simulink model "Assignment_2_Final_Submission"  (R2022b)
settings: Solver=FixedStepAuto  StartTime=0.0  StopTime=10.0  FixedStep=1e-3  RelTol=1e-3  EnableMultiTasking=on
undefined symbols (not defined in the file): A0, A1, D0, D1, D10, D11, D12, D13, D2, D3, D4, D5, D6, D7, D8, D9, magnitude, PTA0, PTA1, PTA2, PTB2, PTB23, PTB3, PTB9, PTC16, PTC17, PTC2, PTC3, PTC4, PTD0, PTD1, PTD2, PTD3
libraries: frdmk64flib x19, etargetslib x8, simulink x2, dspstat3 x1
(part 1 of 2)
settings Model: ExtModeTrigDuration=5  Creator=annan  LastModifiedBy=danie
settings OptimizationCC: EnhancedBackFolding=on  PassReuseOutputArgsAs=Individual arguments  ZeroExternalMemoryAtStartup=off  ZeroInternalMemoryAtStartup=off  MaxStackSize=64  OptimizeBlockOrder=speed  DifferentSizesBufferReuse=on  OptimizationCustomize=off  EfficientTunableParamExpr=on
settings DebuggingCC: ParameterTunabilityLossMsg=error
settings HardwareCC: ProdBitPerPointer=32  ProdBitPerSizeT=32  ProdBitPerPtrDiffT=32  ProdLargestAtomicInteger=Long  ProdLargestAtomicFloat=Double  ProdWordSize=32  ProdHWDeviceType=ARM Compatible->ARM Cortex
settings SFSimCC: MATLABDynamicMemAlloc=off
settings RTWCC: Description=Embedded Coder  SystemTargetFile=ert.tlc  HardwareBoard=NXP FRDM-K64F  TLCOptions="-aInlineSetEventsForThisBaseRateFcn=TLC_FALSE -aSuppressMultiTaskScheduler=TLC_FALSE  -aRateBasedStepFcn=0"  TemplateMakefile=ert_default_tmf  Toolchain=GNU Tools for ARM Embedded Processors
settings CodeAppCC: ForceParamTrailComments=on  IgnoreCustomStorageClasses=off  OperatorAnnotations=on  SimulinkDataObjDesc=on  SFDataObjDesc=on  InsertBlockDesc=on
settings ERTTargetCC: ExtModeTransport=4  ExtModeMexFile=sendToCommService

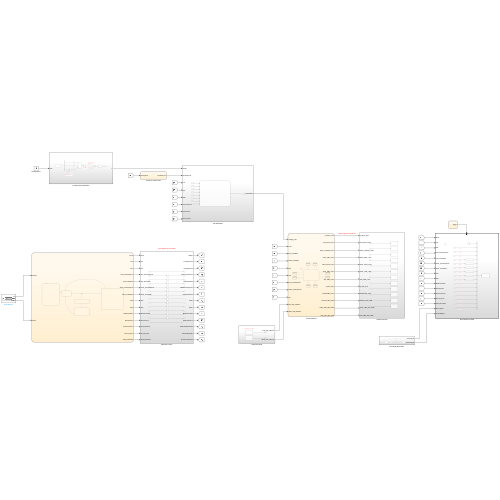
[thumbnail: Simulink's stored preview of the top-level diagram]
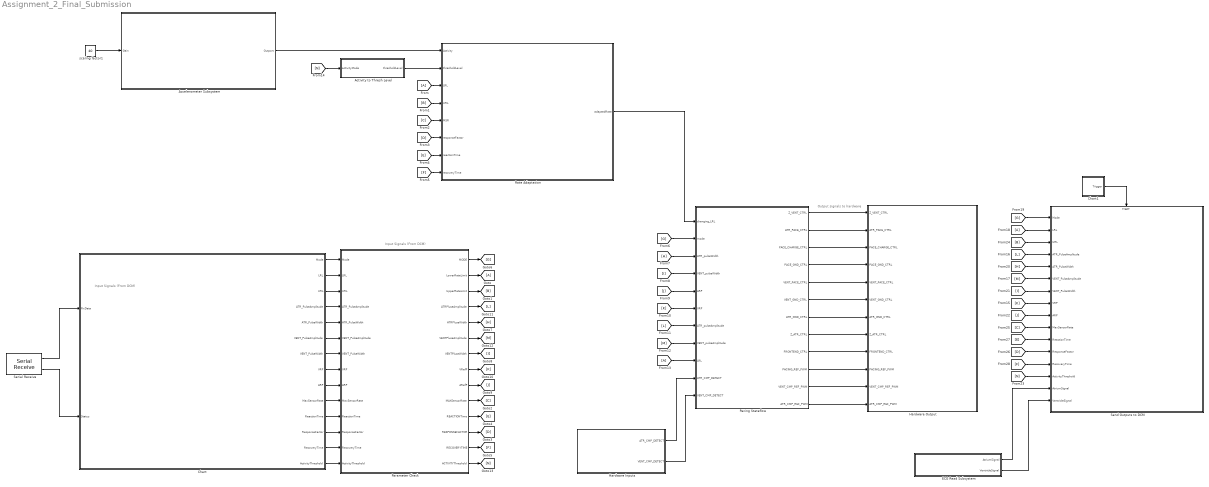
== system Assignment_2_Final_Submission ==
  note: Input Signals (From DCM)
  note: Output signals to hardware
  note: Input Signals (From DCM)
  Accelerometer Subsystem : Subsystem
  Activity to Thresh Level : Stateflow chart  TreatAsAtomicUnit=on
  Chart : Stateflow chart  TreatAsAtomicUnit=on
      settings: PortSchema="{\"entries\":[{\"content\":{\"sides\":[{\"content\":{\"connectorIds\":[\"In1\",\"In2\"]},\"type\":\"ConnectorPlacement.EquallySpacedRectSide\",\"uuid\":\"5dec20b2-4828-40f7-ab17-581616d768e4\"},{\"content\":{\"connectorIds\":[\"Out14\",\"Out1\",\"Out13\",\"Out12\",\"Out11\",\"Out10\",\"Out9\",\"Out8\",\"Out7\",\"Out6\",\"Out5\",\"Out4\",\"Out3\",\"Out2\"],\"side\":\"RIGHT\"},\"type\":\"ConnectorPlacement.EquallySpacedRectSide\",\"uuid\":\"fe0d7708-8c60-4078-b2a9-9a22708a989b\"},{\"content\":{\"connectorIds\":[],\"side\":\"TOP\"},\"type\":\"ConnectorPlacement.EquallySpacedRectSide\",\"uuid\":\"c8cd286c-7cc7-4d1d-92dd-859e210849b8\"},{\"content\":{\"connectorIds\":[],\"side\":\"BOTTOM\"},\"type\":\"ConnectorPlacement.EquallySpacedRectSide\",\"uuid\":\"bbfa5a44-a83c-4407-89b4-d26b2a8b5140\"}]},\"type\":\"ConnectorPlacement.EquallySpacedConnector\",\"uuid\":\"7f21e6d2-2aa6-491e-bb3e-ebcef11de234\"}],\"packageUris\":[\"http://schema.mathworks.com/mf0/Connector/R2020b\"],\"version\":\"1.0\"}"
  Chart1 : Stateflow chart  TreatAsAtomicUnit=on
  ECG Read Subsystem : Subsystem
  From : From
  From13 : From
  From18 : From
  Goto : Goto
  Hardware Inputs : Subsystem
  Hardware Output : Subsystem
  Pacing Stateflow : Stateflow chart  TreatAsAtomicUnit=on
      settings: PortSchema="{\"entries\":[{\"content\":{\"sides\":[{\"content\":{\"connectorIds\":[\"In1\",\"In2\",\"In3\",\"In4\",\"In6\",\"In5\",\"In9\",\"In8\",\"In7\",\"In10\",\"In11\"]},\"type\":\"ConnectorPlacement.EquallySpacedRectSide\",\"uuid\":\"576c6451-25f7-4bf9-8ba9-b62bfe0038eb\"},{\"content\":{\"connectorIds\":[\"Out1\",\"Out2\",\"Out3\",\"Out4\",\"Out5\",\"Out6\",\"Out7\",\"Out8\",\"Out9\",\"Out10\",\"Out11\",\"Out12\"],\"side\":\"RIGHT\"},\"type\":\"ConnectorPlacement.EquallySpacedRectSide\",\"uuid\":\"13f5cd1e-83b9-45c9-ae47-e36f7742cdf1\"},{\"content\":{\"connectorIds\":[],\"side\":\"TOP\"},\"type\":\"ConnectorPlacement.EquallySpacedRectSide\",\"uuid\":\"e0eaa1cf-7eb4-4233-8973-4ce0d50eac65\"},{\"content\":{\"connectorIds\":[],\"side\":\"BOTTOM\"},\"type\":\"ConnectorPlacement.EquallySpacedRectSide\",\"uuid\":\"d60b4a6c-f34d-471d-8156-20bbac3fd058\"}]},\"type\":\"ConnectorPlacement.EquallySpacedConnector\",\"uuid\":\"6190d1e8-de04-4ebf-bfa3-72cd0ed3652a\"}],\"packageUris\":[\"http://schema.mathworks.com/mf0/Connector/R2020b\"],\"version\":\"1.0\"}"
  Parameter Check : Subsystem
  Rate Adaptation : Subsystem
  Send Outputs to DCM : Subsystem
  Serial Receive : frdmk64flib/Serial Receive  SCIModule=0  Baudrate=uint32(9600)  Parity=None  StopBits=1  HardwareFlowControl=None  ByteOrder=LittleEndian  DataType=uint8  DataLength=29  BlockingMode=off  OutputStatus=on  SampleTime=-1
  scaling factor1 : Constant  Value=40
  wires:
  Pacing Stateflow/1(Z_VENT_CTRL) -> Hardware Output/1(Z_VENT_CTRL)
  Pacing Stateflow/2(ATR_PACE_CTRL) -> Hardware Output/2(ATR_PACE_CTRL)
  Pacing Stateflow/3(PACE_CHARGE_CTRL) -> Hardware Output/3(PACE_CHARGE_CTRL)
  Pacing Stateflow/4(PACE_GND_CTRL) -> Hardware Output/4(PACE_GND_CTRL)
  Pacing Stateflow/5(VENT_PACE_CTRL) -> Hardware Output/5(VENT_PACE_CTRL)
  Pacing Stateflow/6(VENT_GND_CTRL) -> Hardware Output/6(VENT_GND_CTRL)
  Pacing Stateflow/7(ATR_GND_CTRL) -> Hardware Output/7(ATR_GND_CTRL)
  Pacing Stateflow/8(Z_ATR_CTRL) -> Hardware Output/8(Z_ATR_CTRL)
  From13/1 -> Pacing Stateflow/7(LRL)
  [K] -> Pacing Stateflow/5(VRP)
  [H] -> Pacing Stateflow/3(ATR_pulseWidth)
  Pacing Stateflow/10(PACING_REF_PWM) -> Hardware Output/10(PACING_REF_PWM)
  [M] -> Pacing Stateflow/8(VENT_pulseAmplitude)
  Pacing Stateflow/9(FRONTEND_CTRL) -> Hardware Output/9(FRONTEND_CTRL)
  Pacing Stateflow/11(VENT_CMP_REF_PWM) -> Hardware Output/11(VENT_CMP_REF_PWM)
  Pacing Stateflow/12(ATR_CMP_REF_PWM) -> Hardware Output/12(ATR_CMP_REF_PWM)
  [I] -> Pacing Stateflow/4(VENT_pulseWidth)
  [J] -> Pacing Stateflow/6(ARP)
  [L] -> Pacing Stateflow/9(ATR_pulseAmplitude)
  [G] -> Pacing Stateflow/2(mode)
  [D] -> Rate Adaptation/6(responseFactor)
  [C] -> Rate Adaptation/5(MSR)
  [B] -> Rate Adaptation/4(URL)
  Activity to Thresh Level/1(thresholdLevel) -> Rate Adaptation/2(thresholdLevel)
  Accelerometer Subsystem/1(Outport) -> Rate Adaptation/1(Activity)
  [E] -> Rate Adaptation/7(reactionTime)
  [F] -> Rate Adaptation/8(recoveryTime)
  From/1 -> Rate Adaptation/3(LRL)
  scaling factor1/1 -> Accelerometer Subsystem/1(Gain)
  [N] -> Activity to Thresh Level/1(activityMode)
  Rate Adaptation/1(adaptedRate) -> Pacing Stateflow/1(changing_LRL)
  ECG Read Subsystem/2(VentricleSignal) -> Send Outputs to DCM/16(VentricleSignal)
  ECG Read Subsystem/1(AtriumSignal) -> Send Outputs to DCM/15(AtriumSignal)
  Chart1/1(Trigger) -> Send Outputs to DCM/Trigger
  Hardware Inputs/1(ATR_CMP_DETECT) -> Pacing Stateflow/10(ATR_CMP_DETECT)
  Hardware Inputs/2(VENT_CMP_DETECT) -> Pacing Stateflow/11(VENT_CMP_DETECT)
  Parameter Check/2(LowerRateLimit) -> Goto/1
  Parameter Check/3(UpperRateLimit) -> [B]
  Parameter Check/10(MAXSensorRate) -> [C]
  Parameter Check/12(RESPONSEFACTOR) -> [D]
  Parameter Check/11(REACTIONTime) -> [E]
  Parameter Check/13(RECOVERYTIME) -> [F]
  Parameter Check/1(MODE) -> [G]
  Parameter Check/5(ATRPluseWidth) -> [H]
  Parameter Check/7(VENTPluseWidth) -> [I]
  Parameter Check/9(ARefP) -> [J]
  Parameter Check/8(VRefP) -> [K]
  Parameter Check/4(ATRPluseAmplitude) -> [L]
  Parameter Check/6(VENTPluseAmplitude) -> [M]
  Parameter Check/14(ACTIVITYThreshold) -> [N]
  From18/1 -> Send Outputs to DCM/2(LRL)
  [B] -> Send Outputs to DCM/3(URL)
  [L] -> Send Outputs to DCM/4(ATR_PulseAmplitude)
  [H] -> Send Outputs to DCM/5(ATR_PulseWidth)
  [M] -> Send Outputs to DCM/6(VENT_PulseAmplitude)
  [I] -> Send Outputs to DCM/7(VENT_PulseWidth)
  [G] -> Send Outputs to DCM/1(Mode)
  [K] -> Send Outputs to DCM/8(VRP)
  [J] -> Send Outputs to DCM/9(ARP)
  [C] -> Send Outputs to DCM/10(MaxSensorRate)
  [E] -> Send Outputs to DCM/11(ReactionTime)
  [F] -> Send Outputs to DCM/13(RecoveryTime)
  [D] -> Send Outputs to DCM/12(ResponseFactor)
  Chart/3(RecoveryTime) -> Parameter Check/13("RecoveryTime ")
  Chart/2(ActivityThreshold) -> Parameter Check/14("ActivityThreshold ")
  Chart/7(ARP) -> Parameter Check/9(ARP)
  Chart/10(VENT_PulseAmplitude) -> Parameter Check/6("VENT_PulseAmplitude ")
  Chart/11(ATR_PulseWidth) -> Parameter Check/5("ATR_PulseWidth ")
  Chart/9(VENT_PulseWidth) -> Parameter Check/7("VENT_PulseWidth ")
  Chart/5(ReactionTime) -> Parameter Check/11("ReactionTime ")
  Chart/1(LRL) -> Parameter Check/2(LRL)
  Chart/14(Mode) -> Parameter Check/1(Mode)
  Serial Receive/2 -> Chart/2(Status)
  Serial Receive/1 -> Chart/1(RxData)
  Chart/6(MaxSensorRate) -> Parameter Check/10("MaxSensorRate ")
  Chart/12(ATR_PulseAmplitude) -> Parameter Check/4("ATR_PulseAmplitude ")
  Chart/8(VRP) -> Parameter Check/8(VRP)
  Chart/13(URL) -> Parameter Check/3(URL)
  Chart/4(ResponseFactor) -> Parameter Check/12("ResponseFactor ")
  [N] -> Send Outputs to DCM/14(ActivityThreshold)

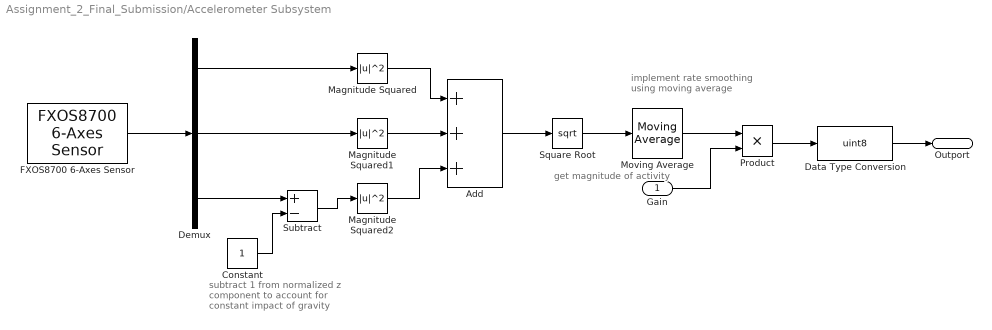
== system Assignment_2_Final_Submission/Accelerometer Subsystem ==
  note: subtract 1 from normalized z component to account for constant impact of gravity
  note: get magnitude of activity
  note: implement rate smoothing using moving average
  Gain : Inport
  Add : Sum  Inputs=+++  OutDataTypeStr=single
  Constant : Constant
  Data Type Conversion : DataTypeConversion  OutDataTypeStr=uint8  SaturateOnIntegerOverflow=off  RndMeth=Floor
  Demux : Demux  Outputs=3
  FXOS8700 6-Axes Sensor : frdmk64flib/FXOS8700 6-Axes Sensor  Activesensor=Accelerometer only  ODR=800Hz  HybridODR=400Hz  Accelfullrange=-4g to +4g  SampleTime=-1
  Magnitude Squared : Math  Operator=magnitude^2  OutDataTypeStr=single
  Magnitude Squared1 : Math  Operator=magnitude^2  OutDataTypeStr=single
  Magnitude Squared2 : Math  Operator=magnitude^2  OutDataTypeStr=single
  Moving Average : dspstat3/Moving Average  Method=Sliding window  ForgettingFactorPort=off  SpecifyWindowLength=on  WindowLength=1  OverlapLength=0  AllowArbitraryInputLength=off  ForgettingFactor=0.9  SimulateUsing=Code generation
  Product : Product
  Square Root : Sqrt  OutDataTypeStr=single
  Subtract : Sum  Inputs=+-
  Outport : Outport  OutDataTypeStr=uint8
  wires:
  FXOS8700 6-Axes Sensor/1 -> Demux/1
  Demux/2 -> Magnitude Squared1/1
  Demux/1 -> Magnitude Squared/1
  Demux/3 -> Subtract/1
  Magnitude Squared2/1 -> Add/3
  Magnitude Squared/1 -> Add/1
  Magnitude Squared1/1 -> Add/2
  Add/1 -> Square Root/1
  Constant/1 -> Subtract/2
  Subtract/1 -> Magnitude Squared2/1
  Square Root/1 -> Moving Average/1
  Gain/1 -> Product/2
  Product/1 -> Data Type Conversion/1
  Data Type Conversion/1 -> Outport/1
  Moving Average/1 -> Product/1

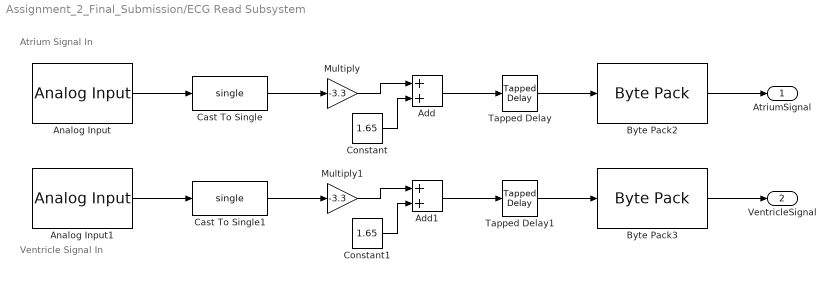
== system Assignment_2_Final_Submission/ECG Read Subsystem ==
  note: Ventricle Signal In
  note: Atrium Signal In
  Add : Sum
  Add1 : Sum
  Analog Input : frdmk64flib/Analog Input  Whichpin=PTB2 (A0)  SampleTime=0.002
  Analog Input1 : frdmk64flib/Analog Input  Whichpin=PTB3 (A1)  SampleTime=0.002
  Byte Pack2 : etargetslib/Byte Pack  datatypes={'single'}  byteAlign=1
  Byte Pack3 : etargetslib/Byte Pack  datatypes={'single'}  byteAlign=1
  Cast To Single : DataTypeConversion  OutDataTypeStr=single  SaturateOnIntegerOverflow=off  RndMeth=Floor
  Cast To Single1 : DataTypeConversion  OutDataTypeStr=single  SaturateOnIntegerOverflow=off  RndMeth=Floor
  Constant : Constant  Value=1.65  OutDataTypeStr=single
  Constant1 : Constant  Value=1.65  OutDataTypeStr=single
  Multiply : Gain  Gain=-3.3
  Multiply1 : Gain  Gain=-3.3
  Tapped Delay : simulink/Discrete/Tapped Delay  vinit=0.0  samptime=-1  NumDelays=9  DelayOrder=Oldest  includeCurrent=on
  Tapped Delay1 : simulink/Discrete/Tapped Delay  vinit=0.0  samptime=-1  NumDelays=9  DelayOrder=Oldest  includeCurrent=on
  AtriumSignal : Outport
  VentricleSignal : Outport  Port=2
  wires:
  Tapped Delay/1 -> Byte Pack2/1
  Cast To Single1/1 -> Multiply1/1
  Cast To Single/1 -> Multiply/1
  Analog Input/1 -> Cast To Single/1
  Tapped Delay1/1 -> Byte Pack3/1
  Analog Input1/1 -> Cast To Single1/1
  Byte Pack2/1 -> AtriumSignal/1
  Byte Pack3/1 -> VentricleSignal/1
  Add/1 -> Tapped Delay/1
  Multiply/1 -> Add/1
  Constant/1 -> Add/2
  Multiply1/1 -> Add1/1
  Add1/1 -> Tapped Delay1/1
  Constant1/1 -> Add1/2

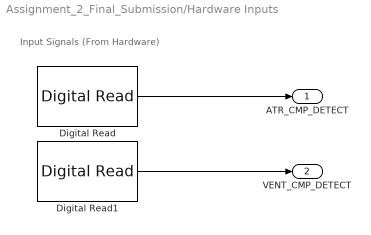
== system Assignment_2_Final_Submission/Hardware Inputs ==
  note: Input Signals (From Hardware)
  Digital Read : frdmk64flib/Digital Read  Whichpin=PTC16 (D0)  SampleTime=-1
  Digital Read1 : frdmk64flib/Digital Read  Whichpin=PTC17 (D1)  SampleTime=-1
  ATR_CMP_DETECT : Outport
  VENT_CMP_DETECT : Outport  Port=2
  wires:
  Digital Read/1 -> ATR_CMP_DETECT/1
  Digital Read1/1 -> VENT_CMP_DETECT/1

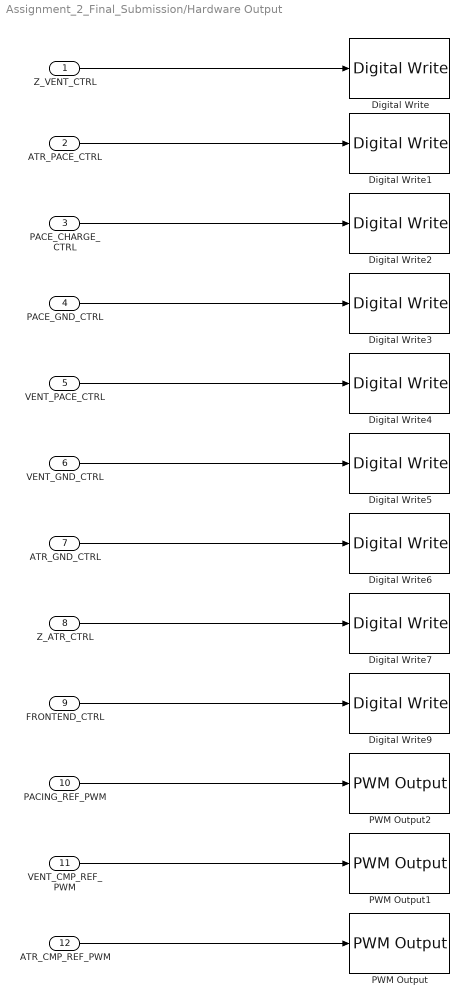
== system Assignment_2_Final_Submission/Hardware Output ==
  Z_VENT_CTRL : Inport
  ATR_PACE_CTRL : Inport  Port=2
  PACE_CHARGE_CTRL : Inport  Port=3
  PACE_GND_CTRL : Inport  Port=4
  VENT_PACE_CTRL : Inport  Port=5
  VENT_GND_CTRL : Inport  Port=6
  ATR_GND_CTRL : Inport  Port=7
  Z_ATR_CTRL : Inport  Port=8
  FRONTEND_CTRL : Inport  Port=9
  PACING_REF_PWM : Inport  Port=10
  VENT_CMP_REF_PWM : Inport  Port=11
  ATR_CMP_REF_PWM : Inport  Port=12
  Digital Write : frdmk64flib/Digital Write  Whichpin=PTC3 (D7)
  Digital Write1 : frdmk64flib/Digital Write  Whichpin=PTA0 (D8)
  Digital Write2 : frdmk64flib/Digital Write  Whichpin=PTB9 (D2)
  Digital Write3 : frdmk64flib/Digital Write  Whichpin=PTD0 (D10)
  Digital Write4 : frdmk64flib/Digital Write  Whichpin=PTC4 (D9)
  Digital Write5 : frdmk64flib/Digital Write  Whichpin=PTD3 (D12)
  Digital Write6 : frdmk64flib/Digital Write  Whichpin=PTD2 (D11)
  Digital Write7 : frdmk64flib/Digital Write  Whichpin=PTB23 (D4)
  Digital Write9 : frdmk64flib/Digital Write  Whichpin=PTD1 (D13)
  PWM Output : frdmk64flib/PWM Output  Whichpin=PTC2 (D6)  InitialFrequency=2000  InitialDutyCycle=0
  PWM Output1 : frdmk64flib/PWM Output  Whichpin=PTA1 (D3)  InitialFrequency=2000  InitialDutyCycle=0
  PWM Output2 : frdmk64flib/PWM Output  Whichpin=PTA2 (D5)  InitialFrequency=2000  InitialDutyCycle=0
  wires:
  Z_VENT_CTRL/1 -> Digital Write/1
  ATR_PACE_CTRL/1 -> Digital Write1/1
  PACE_CHARGE_CTRL/1 -> Digital Write2/1
  PACE_GND_CTRL/1 -> Digital Write3/1
  VENT_PACE_CTRL/1 -> Digital Write4/1
  VENT_GND_CTRL/1 -> Digital Write5/1
  ATR_GND_CTRL/1 -> Digital Write6/1
  Z_ATR_CTRL/1 -> Digital Write7/1
  PACING_REF_PWM/1 -> PWM Output2/1
  FRONTEND_CTRL/1 -> Digital Write9/1
  VENT_CMP_REF_PWM/1 -> PWM Output1/1
  ATR_CMP_REF_PWM/1 -> PWM Output/1

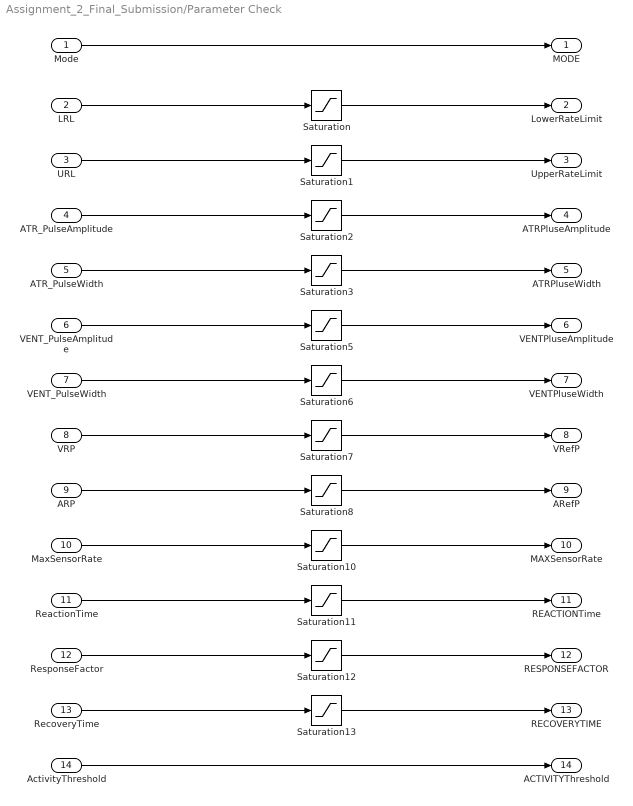
== system Assignment_2_Final_Submission/Parameter Check ==
  Mode : Inport
  LRL : Inport  Port=2
  URL : Inport  Port=3
  "ATR_PulseAmplitude " : Inport  Port=4  OutDataTypeStr=single
  "ATR_PulseWidth " : Inport  Port=5
  "VENT_PulseAmplitude " : Inport  Port=6
  "VENT_PulseWidth " : Inport  Port=7
  VRP : Inport  Port=8
  ARP : Inport  Port=9
  "MaxSensorRate " : Inport  Port=10
  "ReactionTime " : Inport  Port=11
  "ResponseFactor " : Inport  Port=12
  "RecoveryTime " : Inport  Port=13
  "ActivityThreshold " : Inport  Port=14
  Saturation : Saturate  UpperLimit=175  LowerLimit=30
  Saturation1 : Saturate  UpperLimit=175  LowerLimit=60
  Saturation10 : Saturate  UpperLimit=175  LowerLimit=50
  Saturation11 : Saturate  UpperLimit=50  LowerLimit=10
  Saturation12 : Saturate  UpperLimit=16  LowerLimit=1
  Saturation13 : Saturate  UpperLimit=16  LowerLimit=2
  Saturation2 : Saturate  UpperLimit=5  LowerLimit=0.5
  Saturation3 : Saturate  UpperLimit=1.9  LowerLimit=0.05
  Saturation5 : Saturate  UpperLimit=5  LowerLimit=0.5
  Saturation6 : Saturate  UpperLimit=1.9  LowerLimit=0.05
  Saturation7 : Saturate  UpperLimit=500  LowerLimit=150
  Saturation8 : Saturate  UpperLimit=500  LowerLimit=150
  MODE : Outport
  LowerRateLimit : Outport  Port=2
  UpperRateLimit : Outport  Port=3
  ATRPluseAmplitude : Outport  Port=4  OutDataTypeStr=single
  ATRPluseWidth : Outport  Port=5
  VENTPluseAmplitude : Outport  Port=6
  VENTPluseWidth : Outport  Port=7
  VRefP : Outport  Port=8
  ARefP : Outport  Port=9
  MAXSensorRate : Outport  Port=10
  REACTIONTime : Outport  Port=11
  RESPONSEFACTOR : Outport  Port=12
  RECOVERYTIME : Outport  Port=13
  ACTIVITYThreshold : Outport  Port=14
  wires:
  LRL/1 -> Saturation/1
  Saturation/1 -> LowerRateLimit/1
  Saturation1/1 -> UpperRateLimit/1
  URL/1 -> Saturation1/1
  Mode/1 -> MODE/1
  "ATR_PulseAmplitude "/1 -> Saturation2/1
  Saturation2/1 -> ATRPluseAmplitude/1
  "ATR_PulseWidth "/1 -> Saturation3/1
  Saturation3/1 -> ATRPluseWidth/1
  "VENT_PulseAmplitude "/1 -> Saturation5/1
  Saturation5/1 -> VENTPluseAmplitude/1
  "VENT_PulseWidth "/1 -> Saturation6/1
  Saturation6/1 -> VENTPluseWidth/1
  VRP/1 -> Saturation7/1
  Saturation7/1 -> VRefP/1
  ARP/1 -> Saturation8/1
  Saturation8/1 -> ARefP/1
  Saturation10/1 -> MAXSensorRate/1
  "MaxSensorRate "/1 -> Saturation10/1
  Saturation11/1 -> REACTIONTime/1
  "ReactionTime "/1 -> Saturation11/1
  Saturation12/1 -> RESPONSEFACTOR/1
  "ResponseFactor "/1 -> Saturation12/1
  Saturation13/1 -> RECOVERYTIME/1
  "RecoveryTime "/1 -> Saturation13/1
  "ActivityThreshold "/1 -> ACTIVITYThreshold/1

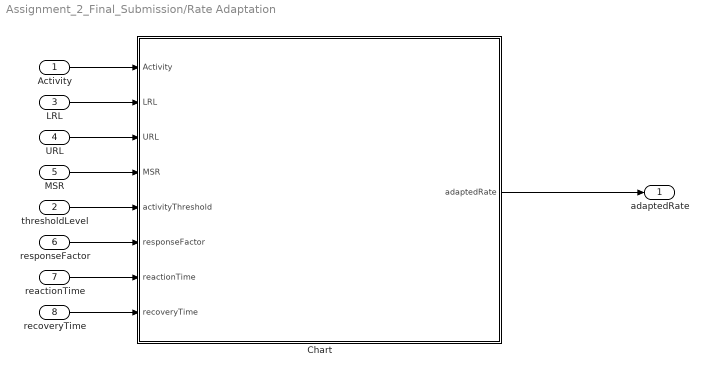
== system Assignment_2_Final_Submission/Rate Adaptation ==
  Activity : Inport  OutDataTypeStr=uint8
  thresholdLevel : Inport  Port=2
  LRL : Inport  Port=3  OutDataTypeStr=uint8
  URL : Inport  Port=4  OutDataTypeStr=uint8
  MSR : Inport  Port=5
  responseFactor : Inport  Port=6
  reactionTime : Inport  Port=7
  recoveryTime : Inport  Port=8
  Chart : Stateflow chart  TreatAsAtomicUnit=on
  adaptedRate : Outport
  wires:
  Activity/1 -> Chart/1(Activity)
  LRL/1 -> Chart/2(LRL)
  URL/1 -> Chart/3(URL)
  MSR/1 -> Chart/4(MSR)
  thresholdLevel/1 -> Chart/5(activityThreshold)
  responseFactor/1 -> Chart/6(responseFactor)
  reactionTime/1 -> Chart/7(reactionTime)
  recoveryTime/1 -> Chart/8(recoveryTime)
  Chart/1(adaptedRate) -> adaptedRate/1

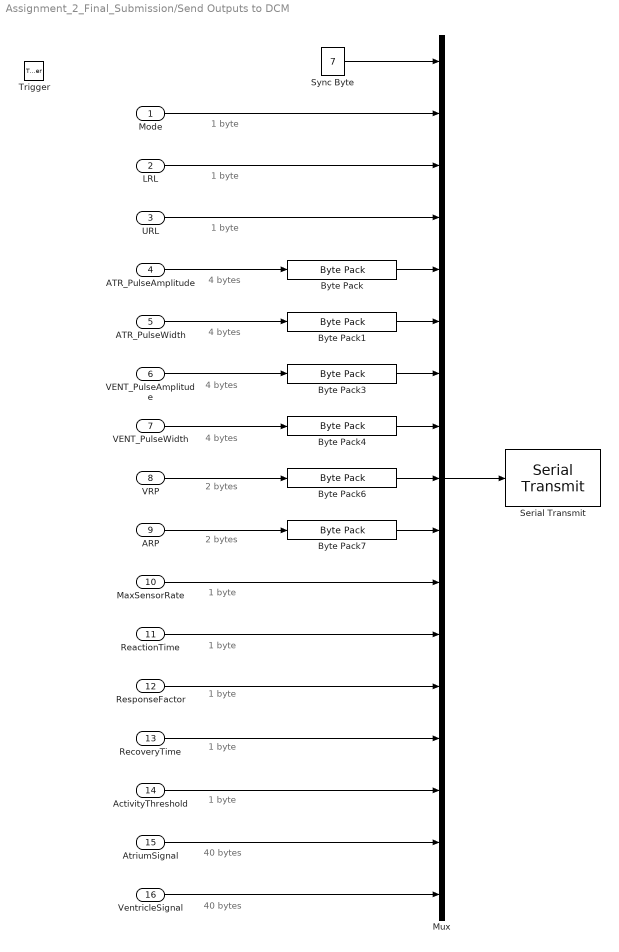
== system Assignment_2_Final_Submission/Send Outputs to DCM ==
  note: 40 bytes
  note: 1 byte
  note: 1 byte
  note: 1 byte
  note: 4 bytes
  note: 4 bytes
  note: 4 bytes
  note: 4 bytes
  note: 2 bytes
  note: 2 bytes
  note: 1 byte
  note: 1 byte
  note: 1 byte
  note: 1 byte
  note: 1 byte
  note: 40 bytes
  Mode : Inport
  LRL : Inport  Port=2
  URL : Inport  Port=3
  ATR_PulseAmplitude : Inport  Port=4  OutDataTypeStr=single
  ATR_PulseWidth : Inport  Port=5  OutDataTypeStr=single
  VENT_PulseAmplitude : Inport  Port=6
  VENT_PulseWidth : Inport  Port=7
  VRP : Inport  Port=8
  ARP : Inport  Port=9
  MaxSensorRate : Inport  Port=10
  ReactionTime : Inport  Port=11
  ResponseFactor : Inport  Port=12
  RecoveryTime : Inport  Port=13
  ActivityThreshold : Inport  Port=14
  AtriumSignal : Inport  Port=15
  VentricleSignal : Inport  Port=16
  Trigger : TriggerPort  FunctionName=UART_Tx  VariantControl=(inherit)  PortDimensions=1
  Byte Pack{,1,3..4} (4 alike) : etargetslib/Byte Pack  datatypes={'single'}  byteAlign=1
  Byte Pack6 : etargetslib/Byte Pack  datatypes={'uint16'}  byteAlign=1
  Byte Pack7 : etargetslib/Byte Pack  datatypes={'uint16'}  byteAlign=1
  Mux : Mux  Inputs=17
  Serial Transmit : frdmk64flib/Serial Transmit  SCIModule=0  Baudrate=uint32(9600)  Parity=None  StopBits=1  HardwareFlowControl=None  ByteOrder=LittleEndian  BlockingMode=off  OutputStatus=off
  Sync Byte : Constant  Value=7  OutDataTypeStr=uint8
  wires:
  Mux/1 -> Serial Transmit/1
  ATR_PulseAmplitude/1 -> Byte Pack/1
  ATR_PulseWidth/1 -> Byte Pack1/1
  VENT_PulseAmplitude/1 -> Byte Pack3/1
  VENT_PulseWidth/1 -> Byte Pack4/1
  VRP/1 -> Byte Pack6/1
  ARP/1 -> Byte Pack7/1
  Byte Pack3/1 -> Mux/7
  Byte Pack4/1 -> Mux/8
  Byte Pack6/1 -> Mux/9
  Byte Pack7/1 -> Mux/10
  MaxSensorRate/1 -> Mux/11
  ReactionTime/1 -> Mux/12
  ResponseFactor/1 -> Mux/13
  Byte Pack1/1 -> Mux/6
  Byte Pack/1 -> Mux/5
  URL/1 -> Mux/4
  LRL/1 -> Mux/3
  Mode/1 -> Mux/2
  Sync Byte/1 -> Mux/1
  ActivityThreshold/1 -> Mux/15
  AtriumSignal/1 -> Mux/16
  VentricleSignal/1 -> Mux/17
  RecoveryTime/1 -> Mux/14

== stateflow chart Assignment_2_Final_Submission/Activity to Thresh Level ==
  state Activity_to_Threshold
    entry:
    %very low
    if activityMode == 0
    thresholdLevel = 20;
    end
    %low
    if activityMode == 1
    thresholdLevel = 40;
    end
    %med low
    if activityMode == 2
    thresholdLevel = 60;
    end
    %med
    if activityMode == 3
    thresholdLevel = 80;
    end
    %med high
    if activityMode == 4
    thresholdLevel = 100;
    end
    %high
    if activityMode == 5
    thresholdLevel = 120;
    end
    %very high
    if activityMode == 6
    thresholdLevel = 140;
    end
  (default) -> Activity_to_Threshold
  Activity_to_Threshold -> Activity_to_Threshold
  data: thresholdLevel output uint8; activityMode input uint8

== stateflow chart Assignment_2_Final_Submission/Chart ==
  settings: executeAtInitialization=1
  note: A default of parameters that does not depend on DCM input.
  note: SettingParameters block is used to typecast the parameters that are used in the main stateflow of the pacemaker. The data within the parameters are created and sent from the DCM.
  state Init
    entry:
    %Default parameters set
    Mode = 1;
    LRL = 60;
    URL = 120;
    ATR_PulseAmplitude = 3.5;
    ATR_PulseWidth = 0.4;
    VENT_PulseAmplitude = 3.5;
    VENT_PulseWidth = 0.4;
    ARP = 250;
    VRP = 320;
    MaxSensorRate = 120;
    ReactionTime = 30;
    ResponseFactor = 8;
    RecoveryTime = 5;
    ActivityThreshold = 3;
  state SettingParameters
    entry:
    Mode = RxData(2);
    LRL = RxData(3);
    URL = RxData(4);
    ATR_PulseAmplitude = typecast(RxData(5:8), "single");
    ATR_PulseWidth = typecast(RxData(9:12),"single");
    VENT_PulseAmplitude = typecast(RxData(13:16), "single");
    VENT_PulseWidth = typecast(RxData(17:20),"single");
    VRP = typecast(RxData(21:22),"uint16");
    ARP = typecast(RxData(23:24),"uint16");
    MaxSensorRate = RxData(25);
    ReactionTime = RxData(26);
    ResponseFactor = RxData(27);
    RecoveryTime = RxData(28);
    ActivityThreshold = RxData(29);
  state Stall
    entry:
  state WaitForBuffer
    %Waits for new values for the Buffer
  state SendECG
  SettingParameters -> Stall
  (default) -> Init
  Init -> Stall
  Stall -> (junction 7) : [Status == 0]
  (junction 7) -> SettingParameters [order 2]
  (junction 7) -> WaitForBuffer [order 1] : [RxData(1) == hex2dec('55')]
  SendECG -> Stall
  WaitForBuffer -> SendECG : [after(20,msec)]
  data: LRL output uint8; ActivityThreshold output uint8; RecoveryTime output uint8; ResponseFactor output uint8; ReactionTime output uint8; MaxSensorRate output uint8; ARP output uint16; VRP output uint16; VENT_PulseWidth output single; VENT_PulseAmplitude output single; ATR_PulseWidth output single; ATR_PulseAmplitude output single; URL output uint8; RxData input uint8 size=29; Status input uint8 size=1; Mode output uint8
